simulink model "mesaparasimulink"  (R2017a)
settings: Solver=ode3  StartTime=0.0  StopTime=6.3  FixedStep=5e-3  RelTol=1e-3
undefined symbols (not defined in the file): bloque, bloque1, L1, L2, mesaparasimulink, pasador, RootGround, RootPart
libraries: mblibv1 x24
settings Model: Creator=angel  LastModifiedBy=angel
settings SimMechanicsCC: VisOnUpdateDiagram=on  VisDuringSimulation=on

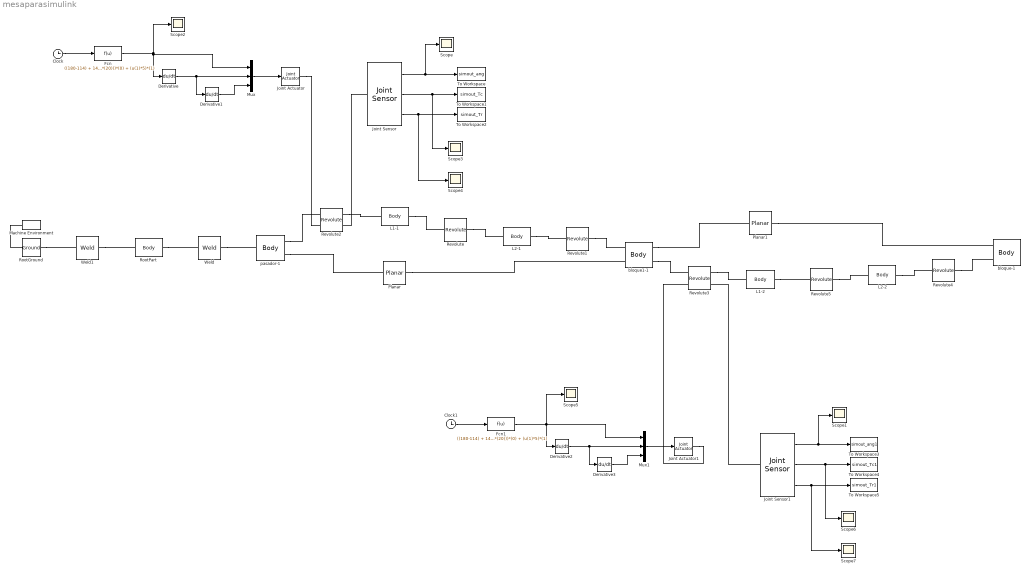
== system mesaparasimulink ==
  Clock : Clock
  Clock1 : Clock
  Derivative{,1..3} (4 alike) : Derivative
  Fcn : Fcn  Expr=((180-114) + 14*sin(2*pi*u(1)*(20)))*(0) + (u(1)*5)*(1)
  Fcn1 : Fcn  Expr=((180-114) + 14*sin(2*pi*u(1)*(20)))*(0) + (u(1)*5)*(1)
  Joint Actuator : mblibv1/Sensors &  Actuators/Joint Actuator  UpdateFromCAD=off  PhysicalDomain=Mechanical  PortType=blob  ActuationStyle=Motion  AngleUnits=rad  ArcVelocityUnits=rad/s  ArcAccelerationUnits=rad/s^2  CoordPositionUnits=m  VelocityUnits=m/s  AccelerationUnits=m/s^2  ForceUnits=N  TorqueUnits=N*m  ActiveIO=on  Width=3  DialogClass=MechanicalActuatorBlock  Primitive=R1  ReferenceFrame=Absolute (World)
      settings: SourceProductName=Simscape Multibody  SourceProductBaseCode=MS
  Joint Actuator1 : mblibv1/Sensors &  Actuators/Joint Actuator  UpdateFromCAD=off  PhysicalDomain=Mechanical  PortType=blob  ActuationStyle=Motion  AngleUnits=rad  ArcVelocityUnits=rad/s  ArcAccelerationUnits=rad/s^2  CoordPositionUnits=m  VelocityUnits=m/s  AccelerationUnits=m/s^2  ForceUnits=N  TorqueUnits=N*m  ActiveIO=on  Width=3  DialogClass=MechanicalActuatorBlock  Primitive=R1  ReferenceFrame=Absolute (World)
      settings: SourceProductName=Simscape Multibody  SourceProductBaseCode=MS
  Joint Sensor : mblibv1/Sensors &  Actuators/Joint Sensor  UpdateFromCAD=off  PhysicalDomain=Mechanical  PortType=blob  Muxed=off  Pose=off  Angle=on  AngleUnits=deg  ArcVelocity=off  ArcVelocityUnits=deg/s  ArcAcceleration=off  ArcAccelerationUnits=deg/s^2  CoordPosition=on  CoordPositionUnits=m  Velocity=off  VelocityUnits=m/s  Acceleration=off  AccelerationUnits=m/s^2  Quaternion=on  QuaternionDT=off  QuaternionDDT=off  QuaternionUnits=off  OutputVector=[1]  ActiveIO=on  Width=5  DialogClass=MechanicalSensorBlock  Primitive=R1  Force=off  ForceUnits=N  Torque=on  TorqueUnits=N*m  ReferenceFrame=Absolute (World)  ReactionSensedSide=Base  ReactionReferenceFrame=Absolute (World)  ReactionForce=off  ReactionForceUnits=N  ReactionMoment=on  ReactionMomentUnits=N*m
      settings: SourceProductName=Simscape Multibody  SourceProductBaseCode=MS
  Joint Sensor1 : mblibv1/Sensors &  Actuators/Joint Sensor  UpdateFromCAD=off  PhysicalDomain=Mechanical  PortType=blob  Muxed=off  Pose=off  Angle=on  AngleUnits=deg  ArcVelocity=off  ArcVelocityUnits=deg/s  ArcAcceleration=off  ArcAccelerationUnits=deg/s^2  CoordPosition=on  CoordPositionUnits=m  Velocity=off  VelocityUnits=m/s  Acceleration=off  AccelerationUnits=m/s^2  Quaternion=on  QuaternionDT=off  QuaternionDDT=off  QuaternionUnits=off  OutputVector=[1]  ActiveIO=on  Width=5  DialogClass=MechanicalSensorBlock  Primitive=R1  Force=off  ForceUnits=N  Torque=on  TorqueUnits=N*m  ReferenceFrame=Absolute (World)  ReactionSensedSide=Base  ReactionReferenceFrame=Absolute (World)  ReactionForce=off  ReactionForceUnits=N  ReactionMoment=on  ReactionMomentUnits=N*m
      settings: SourceProductName=Simscape Multibody  SourceProductBaseCode=MS
  L1-1 : mblibv1/Bodies/Body  LConnTagsString=CS3  RConnTagsString=CS2  UpdateFromCAD=on  PMImportedID=L1-1  DialogClass=MechanicalBodyBlock  Mass=0.00593014  MassUnits=kg  InertiaUnits=kg*m^2  Inertia=[1.04021e-06,0,0;0,1.07865e-06,0;0,0,6.31529e-08]  Shape=Cylinder  ShapeDims=[1 1]  ShapeUnits=m  ShapeUse=false  Density=1  DensityUnits=kg/m^3  DensityUse=false  GraphicsMode=GFXFILE  GraphicsFileName=mesaparasimulink - L1-1.STL  BodyColorSelMode=COLORPALETTE  BodyColor=[0.898039;0.917647;0.929412]  AttachedToCS=CS1  CG=Right$CG$[0.017646 0.00118407 -0.000436433]$WORLD$WORLD$m$[0.521822 0 -0.853055;0 1 0;0.853055 0 0.521822]$3x3 Transform$rad$WORLD$false$L1-1::CG(AUTOGEN)  WorkingFrames=Right$CS1$[0.00058486 -0.00131593 0.01]$WORLD$WORLD$m$[0.521822 0 -0.853055;0 1 0;0.853055 0 0.521822]$3x3 Transform$rad$WORLD$false$L1-1::CS1(AUTOGEN)#Right$CS2$[0.034707 0.00368407 -0.0108729]$WORLD$WORLD$m$[1 0 0;0 1 0;0 0 1]$3x3 Transform$rad$WORLD$true$L1-1:-:L2-1::L1-1(AUTOGEN)#Left$CS3$[0.00058486 0.00368407 0.01]$WORLD$WORLD$m$[1 0 0;0 1 0;0 0 1]$3x3 Transform$rad$WORLD$true$L1-1:-:pasador-1::L1-1(AUTOGEN)  CGPos=[0.017646 0.00118407 -0.000436433]  CGRot=[0.521822 0 -0.853055;0 1 0;0.853055 0 0.521822]  CS0Pos=[]  CS0Rot=[]  CS1Pos=[0.00058486 -0.00131593 0.01]  CS1Rot=[0.521822 0 -0.853055;0 1 0;0.853055 0 0.521822]  CS2Pos=[0.034707 0.00368407 -0.0108729]  CS2Rot=[1 0 0;0 1 0;0 0 1]  CS3Pos=[0.00058486 0.00368407 0.01]  CS3Rot=[1 0 0;0 1 0;0 0 1]  CS4Pos=[]  CS4Rot=[]  CS5Pos=[]  CS5Rot=[]  CS6Pos=[]  CS6Rot=[]  CS7Pos=[]  CS7Rot=[]  CS8Pos=[]  CS8Rot=[]  CS9Pos=[]  CS9Rot=[]  CS10Pos=[]  CS10Rot=[]  CS11Pos=[]  CS11Rot=[]  CS12Pos=[]  CS12Rot=[]  CS13Pos=[]  CS13Rot=[]  CS14Pos=[]  CS14Rot=[]  CS15Pos=[]  CS15Rot=[]  CS16Pos=[]  CS16Rot=[]  CS17Pos=[]  CS17Rot=[]  CS18Pos=[]  CS18Rot=[]  CS19Pos=[]  CS19Rot=[]  CS20Pos=[]  CS20Rot=[]
      settings: SourceProductName=Simscape Multibody  SourceProductBaseCode=MS
  L1-2 : mblibv1/Bodies/Body  LConnTagsString=CS2  RConnTagsString=CS3  UpdateFromCAD=on  PMImportedID=L1-2  DialogClass=MechanicalBodyBlock  Mass=0.00593014  MassUnits=kg  InertiaUnits=kg*m^2  Inertia=[1.04021e-06,0,0;0,1.07865e-06,0;0,0,6.31529e-08]  Shape=Cylinder  ShapeDims=[1 1]  ShapeUnits=m  ShapeUse=false  Density=1  DensityUnits=kg/m^3  DensityUse=false  GraphicsMode=GFXFILE  GraphicsFileName=mesaparasimulink - L1-2.STL  BodyColorSelMode=COLORPALETTE  BodyColor=[0.898039;0.917647;0.929412]  AttachedToCS=CS1  CG=Right$CG$[0.226845 0.0339841 -0.261953]$WORLD$WORLD$m$[0.998014 0 -0.0629932;0 1 0;0.0629932 0 0.998014]$3x3 Transform$rad$WORLD$false$L1-2::CG(AUTOGEN)  WorkingFrames=Right$CS1$[0.225585 0.0314841 -0.241993]$WORLD$WORLD$m$[0.998014 0 -0.0629932;0 1 0;0.0629932 0 0.998014]$3x3 Transform$rad$WORLD$false$L1-2::CS1(AUTOGEN)#Left$CS2$[0.225585 0.0364841 -0.241993]$WORLD$WORLD$m$[1 0 0;0 1 0;0 0 1]$3x3 Transform$rad$WORLD$true$L1-2:-:bloque1-1::L1-2(AUTOGEN)#Right$CS3$[0.228105 0.0364841 -0.281914]$WORLD$WORLD$m$[1 0 0;0 1 0;0 0 1]$3x3 Transform$rad$WORLD$true$L1-2:-:L2-2::L1-2(AUTOGEN)  CGPos=[0.226845 0.0339841 -0.261953]  CGRot=[0.998014 0 -0.0629932;0 1 0;0.0629932 0 0.998014]  CS0Pos=[]  CS0Rot=[]  CS1Pos=[0.225585 0.0314841 -0.241993]  CS1Rot=[0.998014 0 -0.0629932;0 1 0;0.0629932 0 0.998014]  CS2Pos=[0.225585 0.0364841 -0.241993]  CS2Rot=[1 0 0;0 1 0;0 0 1]  CS3Pos=[0.228105 0.0364841 -0.281914]  CS3Rot=[1 0 0;0 1 0;0 0 1]  CS4Pos=[]  CS4Rot=[]  CS5Pos=[]  CS5Rot=[]  CS6Pos=[]  CS6Rot=[]  CS7Pos=[]  CS7Rot=[]  CS8Pos=[]  CS8Rot=[]  CS9Pos=[]  CS9Rot=[]  CS10Pos=[]  CS10Rot=[]  CS11Pos=[]  CS11Rot=[]  CS12Pos=[]  CS12Rot=[]  CS13Pos=[]  CS13Rot=[]  CS14Pos=[]  CS14Rot=[]  CS15Pos=[]  CS15Rot=[]  CS16Pos=[]  CS16Rot=[]  CS17Pos=[]  CS17Rot=[]  CS18Pos=[]  CS18Rot=[]  CS19Pos=[]  CS19Rot=[]  CS20Pos=[]  CS20Rot=[]
      settings: SourceProductName=Simscape Multibody  SourceProductBaseCode=MS
  L2-1 : mblibv1/Bodies/Body  LConnTagsString=CS2  RConnTagsString=CS3  UpdateFromCAD=on  PMImportedID=L2-1  DialogClass=MechanicalBodyBlock  Mass=0.00998014  MassUnits=kg  InertiaUnits=kg*m^2  Inertia=[4.69227e-06,0,0;0,4.75602e-06,0;0,0,1.0534e-07]  Shape=Cylinder  ShapeDims=[1 1]  ShapeUnits=m  ShapeUse=false  Density=1  DensityUnits=kg/m^3  DensityUse=false  GraphicsMode=GFXFILE  GraphicsFileName=mesaparasimulink - L2-1.STL  BodyColorSelMode=COLORPALETTE  BodyColor=[0.898039;0.917647;0.929412]  AttachedToCS=CS1  CG=Right$CG$[0.017646 0.00618407 -0.041433]$WORLD$WORLD$m$[0.873145 0 0.48746;0 1 0;-0.48746 0 0.873145]$3x3 Transform$rad$WORLD$false$L2-1::CG(AUTOGEN)  WorkingFrames=Right$CS1$[0.034707 0.00368407 -0.0108729]$WORLD$WORLD$m$[0.873145 0 0.48746;0 1 0;-0.48746 0 0.873145]$3x3 Transform$rad$WORLD$false$L2-1::CS1(AUTOGEN)#Left$CS2$[0.034707 0.00368407 -0.0108729]$WORLD$WORLD$m$[1 0 0;0 1 0;0 0 1]$3x3 Transform$rad$WORLD$true$L1-1:-:L2-1::L2-1(AUTOGEN)#Right$CS3$[0.00058486 0.00368407 -0.071993]$WORLD$WORLD$m$[1 0 0;0 1 0;0 0 1]$3x3 Transform$rad$WORLD$true$L2-1:-:bloque1-1::L2-1(AUTOGEN)  CGPos=[0.017646 0.00618407 -0.041433]  CGRot=[0.873145 0 0.48746;0 1 0;-0.48746 0 0.873145]  CS0Pos=[]  CS0Rot=[]  CS1Pos=[0.034707 0.00368407 -0.0108729]  CS1Rot=[0.873145 0 0.48746;0 1 0;-0.48746 0 0.873145]  CS2Pos=[0.034707 0.00368407 -0.0108729]  CS2Rot=[1 0 0;0 1 0;0 0 1]  CS3Pos=[0.00058486 0.00368407 -0.071993]  CS3Rot=[1 0 0;0 1 0;0 0 1]  CS4Pos=[]  CS4Rot=[]  CS5Pos=[]  CS5Rot=[]  CS6Pos=[]  CS6Rot=[]  CS7Pos=[]  CS7Rot=[]  CS8Pos=[]  CS8Rot=[]  CS9Pos=[]  CS9Rot=[]  CS10Pos=[]  CS10Rot=[]  CS11Pos=[]  CS11Rot=[]  CS12Pos=[]  CS12Rot=[]  CS13Pos=[]  CS13Rot=[]  CS14Pos=[]  CS14Rot=[]  CS15Pos=[]  CS15Rot=[]  CS16Pos=[]  CS16Rot=[]  CS17Pos=[]  CS17Rot=[]  CS18Pos=[]  CS18Rot=[]  CS19Pos=[]  CS19Rot=[]  CS20Pos=[]  CS20Rot=[]
      settings: SourceProductName=Simscape Multibody  SourceProductBaseCode=MS
  L2-2 : mblibv1/Bodies/Body  LConnTagsString=CS3  RConnTagsString=CS2  UpdateFromCAD=on  PMImportedID=L2-2  DialogClass=MechanicalBodyBlock  Mass=0.00998014  MassUnits=kg  InertiaUnits=kg*m^2  Inertia=[4.69227e-06,0,0;0,4.75602e-06,0;0,0,1.0534e-07]  Shape=Cylinder  ShapeDims=[1 1]  ShapeUnits=m  ShapeUse=false  Density=1  DensityUnits=kg/m^3  DensityUse=false  GraphicsMode=GFXFILE  GraphicsFileName=mesaparasimulink - L2-2.STL  BodyColorSelMode=COLORPALETTE  BodyColor=[0.898039;0.917647;0.929412]  AttachedToCS=CS1  CG=Right$CG$[0.199354 0.0389841 -0.261953]$WORLD$WORLD$m$[-0.570294 0 0.821441;0 1 0;-0.821441 0 -0.570294]$3x3 Transform$rad$WORLD$false$L2-2::CG(AUTOGEN)  WorkingFrames=Right$CS1$[0.228105 0.0364841 -0.281914]$WORLD$WORLD$m$[-0.570294 0 0.821441;0 1 0;-0.821441 0 -0.570294]$3x3 Transform$rad$WORLD$false$L2-2::CS1(AUTOGEN)#Right$CS2$[0.170604 0.0414841 -0.241993]$WORLD$WORLD$m$[1 0 0;0 1 0;0 0 1]$3x3 Transform$rad$WORLD$true$L2-2:-:bloque-1::L2-2(AUTOGEN)#Left$CS3$[0.228105 0.0364841 -0.281914]$WORLD$WORLD$m$[1 0 0;0 1 0;0 0 1]$3x3 Transform$rad$WORLD$true$L1-2:-:L2-2::L2-2(AUTOGEN)  CGPos=[0.199354 0.0389841 -0.261953]  CGRot=[-0.570294 0 0.821441;0 1 0;-0.821441 0 -0.570294]  CS0Pos=[]  CS0Rot=[]  CS1Pos=[0.228105 0.0364841 -0.281914]  CS1Rot=[-0.570294 0 0.821441;0 1 0;-0.821441 0 -0.570294]  CS2Pos=[0.170604 0.0414841 -0.241993]  CS2Rot=[1 0 0;0 1 0;0 0 1]  CS3Pos=[0.228105 0.0364841 -0.281914]  CS3Rot=[1 0 0;0 1 0;0 0 1]  CS4Pos=[]  CS4Rot=[]  CS5Pos=[]  CS5Rot=[]  CS6Pos=[]  CS6Rot=[]  CS7Pos=[]  CS7Rot=[]  CS8Pos=[]  CS8Rot=[]  CS9Pos=[]  CS9Rot=[]  CS10Pos=[]  CS10Rot=[]  CS11Pos=[]  CS11Rot=[]  CS12Pos=[]  CS12Rot=[]  CS13Pos=[]  CS13Rot=[]  CS14Pos=[]  CS14Rot=[]  CS15Pos=[]  CS15Rot=[]  CS16Pos=[]  CS16Rot=[]  CS17Pos=[]  CS17Rot=[]  CS18Pos=[]  CS18Rot=[]  CS19Pos=[]  CS19Rot=[]  CS20Pos=[]  CS20Rot=[]
      settings: SourceProductName=Simscape Multibody  SourceProductBaseCode=MS
  Machine Environment : mblibv1/Bodies/Machine Environment  PortType=env  PhysicalDomain=Mechanical  DialogTemplateClass=MECH.MachineEnvironment  SyncWhenCopied=off  Gravity=[0 -9.81 0]  GravityUnits=m/s^2  GravityAsSignal=off  Dimensionality=Auto-detect  AnalysisType=Forward dynamics  LinearAssemblyTolerance=1e-3  LinearAssemblyToleranceUnits=m  AngularAssemblyTolerance=1e-3  AngularAssemblyToleranceUnits=rad  ConstraintSolverType=Stabilizing  ConstraintRelTolerance=1e-4  ConstraintAbsTolerance=1e-4  UseRobustSingularityHandling=off  RedundancyAnalysisToleranceType=Automatically select tolerance  RedundancyAnalysisTolerance=1e-14  StatePerturbationType=Fixed  PerturbationSize=1e-5  VisualizeMachine=on  BodyVisualizationType=Use model default body geometries  BodyColorSelMode=Use model default  DefaultBodyColor=[1 0 0]
      settings: SourceProductName=Simscape Multibody  SourceProductBaseCode=MS
  Mux : Mux  Inputs=3
  Mux1 : Mux  Inputs=3
  Planar : mblibv1/Joints/Planar  LConnTagsString=__newl0  RConnTagsString=__newr0  UpdateFromCAD=on  PMImportedID=bloque1-1:-:pasador-1  NumSAPorts=0  CutJoint=off  MarkAsCut=off  Primitives=prismatic_prismatic  PrimitiveProps=P1$WORLD$[0,1,0]$prismatic#P2$WORLD$[0,0,1]$prismatic#R1$WORLD$[-1,0,0]$revolute  DialogClass=JointBlock  P1Axis=[0,1,0]  P2Axis=[0,0,1]  R1Axis=[-1,0,0]
      settings: SourceProductName=Simscape Multibody  SourceProductBaseCode=MS
  Planar1 : mblibv1/Joints/Planar  LConnTagsString=__newl0  RConnTagsString=__newr0  UpdateFromCAD=on  PMImportedID=bloque-1:-:bloque1-1  NumSAPorts=0  CutJoint=off  MarkAsCut=off  Primitives=prismatic_prismatic  PrimitiveProps=P1$WORLD$[1,0,0]$prismatic#P2$WORLD$[0,-1,0]$prismatic#R1$WORLD$[0,0,1]$revolute  DialogClass=JointBlock  P1Axis=[1,0,0]  P2Axis=[0,-1,0]  R1Axis=[0,0,1]
      settings: SourceProductName=Simscape Multibody  SourceProductBaseCode=MS
  Revolute : mblibv1/Joints/Revolute  LConnTagsString=__newl0  RConnTagsString=__newr0  UpdateFromCAD=on  PMImportedID=L1-1:-:L2-1  NumSAPorts=0  CutJoint=off  MarkAsCut=off  Primitives=prismatic  PrimitiveProps=R1$WORLD$[0,1,0]$revolute  DialogClass=JointBlock  R1Axis=[0,1,0]
      settings: SourceProductName=Simscape Multibody  SourceProductBaseCode=MS
  Revolute1 : mblibv1/Joints/Revolute  LConnTagsString=__newl0  RConnTagsString=__newr0  UpdateFromCAD=on  PMImportedID=L2-1:-:bloque1-1  NumSAPorts=0  CutJoint=off  MarkAsCut=off  Primitives=prismatic  PrimitiveProps=R1$WORLD$[0,-1,0]$revolute  DialogClass=JointBlock  R1Axis=[0,-1,0]
      settings: SourceProductName=Simscape Multibody  SourceProductBaseCode=MS
  Revolute2 : mblibv1/Joints/Revolute  LConnTagsString=__newl0|SA1  RConnTagsString=__newr0|SA1  UpdateFromCAD=on  PMImportedID=L1-1:-:pasador-1  NumSAPorts=2  CutJoint=off  MarkAsCut=off  Primitives=prismatic  PrimitiveProps=R1$World$[0,-1,0]$revolute  DialogClass=JointBlock  R1Axis=[0,-1,0]
      settings: SourceProductName=Simscape Multibody  SourceProductBaseCode=MS
  Revolute3 : mblibv1/Joints/Revolute  LConnTagsString=__newl0|SA1  RConnTagsString=__newr0|SA1  UpdateFromCAD=on  PMImportedID=L1-2:-:bloque1-1  NumSAPorts=2  CutJoint=off  MarkAsCut=off  Primitives=prismatic  PrimitiveProps=R1$World$[0,-1,0]$revolute  DialogClass=JointBlock  R1Axis=[0,-1,0]
      settings: SourceProductName=Simscape Multibody  SourceProductBaseCode=MS
  Revolute4 : mblibv1/Joints/Revolute  LConnTagsString=__newl0  RConnTagsString=__newr0  UpdateFromCAD=on  PMImportedID=L2-2:-:bloque-1  NumSAPorts=0  CutJoint=off  MarkAsCut=off  Primitives=prismatic  PrimitiveProps=R1$WORLD$[0,-1,0]$revolute  DialogClass=JointBlock  R1Axis=[0,-1,0]
      settings: SourceProductName=Simscape Multibody  SourceProductBaseCode=MS
  Revolute5 : mblibv1/Joints/Revolute  LConnTagsString=__newl0  RConnTagsString=__newr0  UpdateFromCAD=on  PMImportedID=L1-2:-:L2-2  NumSAPorts=0  CutJoint=off  MarkAsCut=off  Primitives=prismatic  PrimitiveProps=R1$WORLD$[0,1,0]$revolute  DialogClass=JointBlock  R1Axis=[0,1,0]
      settings: SourceProductName=Simscape Multibody  SourceProductBaseCode=MS
  RootGround : mblibv1/Bodies/Ground  UpdateFromCAD=on  PMImportedID=RootGround  LeftPortType=env  RightPortType=workingframe  PhysicalDomain=Mechanical  DialogClass=GroundBlock  CoordPosition=[0.0155003,0.0188998,-0.240245]  CoordPositionUnits=m  StateVectorMgrId=2  MachineId=[3 0]  ShowEnvPort=on  ParameterChecksum=[2085027060, 2068719643, 829486895, 247911722]  TopologyChecksum=[3575472688, 637684525, 4187757033, 1155351781]
      settings: SourceProductName=Simscape Multibody  SourceProductBaseCode=MS
  RootPart : mblibv1/Bodies/Body  LConnTagsString=CS3  RConnTagsString=CS2  UpdateFromCAD=on  PMImportedID=mesaparasimulink/RootPart  DialogClass=MechanicalBodyBlock  Mass=0  MassUnits=kg  InertiaUnits=kg*m^2  Inertia=[0,0,0;0,0,0;0,0,0]  Shape=Cylinder  ShapeDims=[1 1]  ShapeUnits=m  ShapeUse=false  Density=1  DensityUnits=kg/m^3  DensityUse=false  GraphicsMode=MACHINE_DEFAULT  BodyColorSelMode=MACHINE_DEFAULT  BodyColor=[1;0;0]  AttachedToCS=CS1  CG=Right$CG$[0.0155003 0.0188998 -0.240245]$WORLD$WORLD$m$[1 0 0;0 1 0;0 0 1]$3x3 Transform$rad$WORLD$false$mesaparasimulink/RootPart::CG(AUTOGEN)  WorkingFrames=Right$CS1$[0 0 0]$WORLD$WORLD$m$[1 0 0;0 1 0;0 0 1]$3x3 Transform$rad$WORLD$false$mesaparasimulink/RootPart::CS1(AUTOGEN)#Right$CS2$[0.015217 0.00611225 -0.044476]$WORLD$WORLD$m$[1 0 0;0 1 0;0 0 1]$3x3 Transform$rad$WORLD$true$mesaparasimulink/RootPart:-:pasador-1::mesaparasimulink/RootPart(AUTOGEN)#Left$CS3$[0.0155003 0.0188998 -0.240245]$WORLD$WORLD$m$[1 0 0;0 1 0;0 0 1]$3x3 Transform$rad$WORLD$true$RootGround:-:mesaparasimulink/RootPart::mesaparasimulink/RootPart(AUTOGEN)  CGPos=[0.0155003 0.0188998 -0.240245]  CGRot=[1 0 0;0 1 0;0 0 1]  CS0Pos=[]  CS0Rot=[]  CS1Pos=[0 0 0]  CS1Rot=[1 0 0;0 1 0;0 0 1]  CS2Pos=[0.015217 0.00611225 -0.044476]  CS2Rot=[1 0 0;0 1 0;0 0 1]  CS3Pos=[0.0155003 0.0188998 -0.240245]  CS3Rot=[1 0 0;0 1 0;0 0 1]  CS4Pos=[]  CS4Rot=[]  CS5Pos=[]  CS5Rot=[]  CS6Pos=[]  CS6Rot=[]  CS7Pos=[]  CS7Rot=[]  CS8Pos=[]  CS8Rot=[]  CS9Pos=[]  CS9Rot=[]  CS10Pos=[]  CS10Rot=[]  CS11Pos=[]  CS11Rot=[]  CS12Pos=[]  CS12Rot=[]  CS13Pos=[]  CS13Rot=[]  CS14Pos=[]  CS14Rot=[]  CS15Pos=[]  CS15Rot=[]  CS16Pos=[]  CS16Rot=[]  CS17Pos=[]  CS17Rot=[]  CS18Pos=[]  CS18Rot=[]  CS19Pos=[]  CS19Rot=[]  CS20Pos=[]  CS20Rot=[]
      settings: SourceProductName=Simscape Multibody  SourceProductBaseCode=MS
  Scope{,1..7} (8 alike) : Scope
  To Workspace : ToWorkspace  VariableName=simout_ang  SaveFormat=Timeseries  SampleTime=-1
  To Workspace1 : ToWorkspace  VariableName=simout_Tc  SaveFormat=Timeseries  SampleTime=-1
  To Workspace2 : ToWorkspace  VariableName=simout_Tr  SaveFormat=Timeseries  SampleTime=-1
  To Workspace3 : ToWorkspace  VariableName=simout_ang1  SaveFormat=Timeseries  SampleTime=-1
  To Workspace4 : ToWorkspace  VariableName=simout_Tc1  SaveFormat=Timeseries  SampleTime=-1
  To Workspace5 : ToWorkspace  VariableName=simout_Tr1  SaveFormat=Timeseries  SampleTime=-1
  Weld : mblibv1/Joints/Weld  LConnTagsString=__newl0  RConnTagsString=__newr0  UpdateFromCAD=on  PMImportedID=mesaparasimulink/RootPart:-:pasador-1  NumSAPorts=0  CutJoint=off  MarkAsCut=off  Primitives=weld  PrimitiveProps=W$WORLD$[0.57735,0.57735,0.57735]$weld  DialogClass=JointBlock  WAxis=[0.57735,0.57735,0.57735]
      settings: SourceProductName=Simscape Multibody  SourceProductBaseCode=MS
  Weld1 : mblibv1/Joints/Weld  LConnTagsString=__newl0  RConnTagsString=__newr0  UpdateFromCAD=on  PMImportedID=RootGround:-:mesaparasimulink/RootPart  NumSAPorts=0  CutJoint=off  MarkAsCut=off  Primitives=weld  PrimitiveProps=W$WORLD$[0.57735,0.57735,0.57735]$weld  DialogClass=JointBlock  WAxis=[0.57735,0.57735,0.57735]
      settings: SourceProductName=Simscape Multibody  SourceProductBaseCode=MS
  bloque-1 : mblibv1/Bodies/Body  LConnTagsString=CS2|CS3  UpdateFromCAD=on  PMImportedID=bloque-1  DialogClass=MechanicalBodyBlock  Mass=1.38082  MassUnits=kg  InertiaUnits=kg*m^2  Inertia=[0.0207014,0,0;0,0.0416806,0;0,0,0.0211297]  Shape=Cylinder  ShapeDims=[1 1]  ShapeUnits=m  ShapeUse=false  Density=1  DensityUnits=kg/m^3  DensityUse=false  GraphicsMode=GFXFILE  GraphicsFileName=mesaparasimulink - bloque-1.STL  BodyColorSelMode=COLORPALETTE  BodyColor=[0.647059;0.619608;0.588235]  AttachedToCS=CS1  CG=Right$CG$[0.00249192 0.0389841 -0.241993]$WORLD$WORLD$m$[1 0 0;0 1 0;0 0 1]$3x3 Transform$rad$WORLD$false$bloque-1::CG(AUTOGEN)  WorkingFrames=Right$CS1$[0.000603728 0.0389841 -0.241993]$WORLD$WORLD$m$[1 0 0;0 1 0;0 0 1]$3x3 Transform$rad$WORLD$false$bloque-1::CS1(AUTOGEN)#Left$CS2$[0.129445 0.0614841 -0.246993]$WORLD$WORLD$m$[1 0 0;0 1 0;0 0 1]$3x3 Transform$rad$WORLD$true$bloque-1:-:bloque1-1::bloque-1(AUTOGEN)#Left$CS3$[0.170604 0.0414841 -0.241993]$WORLD$WORLD$m$[1 0 0;0 1 0;0 0 1]$3x3 Transform$rad$WORLD$true$L2-2:-:bloque-1::bloque-1(AUTOGEN)  CGPos=[0.00249192 0.0389841 -0.241993]  CGRot=[1 0 0;0 1 0;0 0 1]  CS0Pos=[]  CS0Rot=[]  CS1Pos=[0.000603728 0.0389841 -0.241993]  CS1Rot=[1 0 0;0 1 0;0 0 1]  CS2Pos=[0.129445 0.0614841 -0.246993]  CS2Rot=[1 0 0;0 1 0;0 0 1]  CS3Pos=[0.170604 0.0414841 -0.241993]  CS3Rot=[1 0 0;0 1 0;0 0 1]  CS4Pos=[]  CS4Rot=[]  CS5Pos=[]  CS5Rot=[]  CS6Pos=[]  CS6Rot=[]  CS7Pos=[]  CS7Rot=[]  CS8Pos=[]  CS8Rot=[]  CS9Pos=[]  CS9Rot=[]  CS10Pos=[]  CS10Rot=[]  CS11Pos=[]  CS11Rot=[]  CS12Pos=[]  CS12Rot=[]  CS13Pos=[]  CS13Rot=[]  CS14Pos=[]  CS14Rot=[]  CS15Pos=[]  CS15Rot=[]  CS16Pos=[]  CS16Rot=[]  CS17Pos=[]  CS17Rot=[]  CS18Pos=[]  CS18Rot=[]  CS19Pos=[]  CS19Rot=[]  CS20Pos=[]  CS20Rot=[]
      settings: SourceProductName=Simscape Multibody  SourceProductBaseCode=MS
  bloque1-1 : mblibv1/Bodies/Body  LConnTagsString=CS2|CS3  RConnTagsString=CS4|CS5  UpdateFromCAD=on  PMImportedID=bloque1-1  DialogClass=MechanicalBodyBlock  Mass=2.30927 + (0.7)*(1)  MassUnits=kg  InertiaUnits=kg*m^2  Inertia=[0.0339371,-0.000140996,-0.000492128;-0.000140996,0.0550496,-0.00133315;-0.000492128,-0.00133315,0.0222148]  Shape=Cylinder  ShapeDims=[1 1]  ShapeUnits=m  ShapeUse=false  Density=1  DensityUnits=kg/m^3  DensityUse=false  GraphicsMode=GFXFILE  GraphicsFileName=mesaparasimulink - bloque1-1.STL  BodyColorSelMode=COLORPALETTE  BodyColor=[0.64706 0.61961 0.58823]  AttachedToCS=CS1  CG=Right$CG$[0.021929 0.006979 -0.242263]$WORLD$WORLD$m$[0 0 1;0 1 0;-1 0 0]$3x3 Transform$rad$WORLD$false$bloque1-1::CG(AUTOGEN)  WorkingFrames=Right$CS1$[0.00058486 0.00618407 -0.241993]$WORLD$WORLD$m$[0 0 1;0 1 0;-1 0 0]$3x3 Transform$rad$WORLD$false$bloque1-1::CS1(AUTOGEN)#Left$CS2$[0.00058486 0.00368407 -0.071993]$WORLD$WORLD$m$[1 0 0;0 1 0;0 0 1]$3x3 Transform$rad$WORLD$true$L2-1:-:bloque1-1::bloque1-1(AUTOGEN)#Left$CS3$[0.00558486 0.0186841 -0.0657822]$WORLD$WORLD$m$[1 0 0;0 1 0;0 0 1]$3x3 Transform$rad$WORLD$true$bloque1-1:-:pasador-1::bloque1-1(AUTOGEN)#Right$CS4$[0.129445 0.0614841 -0.246993]$WORLD$WORLD$m$[1 0 0;0 1 0;0 0 1]$3x3 Transform$rad$WORLD$true$bloque-1:-:bloque1-1::bloque1-1(AUTOGEN)#Right$CS5$[0.225585 0.0364841 -0.241993]$WORLD$WORLD$m$[1 0 0;0 1 0;0 0 1]$3x3 Transform$rad$WORLD$true$L1-2:-:bloque1-1::bloque1-1(AUTOGEN)  CGPos=[0.021929 0.006979 -0.242263]  CGRot=[0 0 1;0 1 0;-1 0 0]  CS0Pos=[]  CS0Rot=[]  CS1Pos=[0.00058486 0.00618407 -0.241993]  CS1Rot=[0 0 1;0 1 0;-1 0 0]  CS2Pos=[0.00058486 0.00368407 -0.071993]  CS2Rot=[1 0 0;0 1 0;0 0 1]  CS3Pos=[0.00558486 0.0186841 -0.0657822]  CS3Rot=[1 0 0;0 1 0;0 0 1]  CS4Pos=[0.129445 0.0614841 -0.246993]  CS4Rot=[1 0 0;0 1 0;0 0 1]  CS5Pos=[0.225585 0.0364841 -0.241993]  CS5Rot=[1 0 0;0 1 0;0 0 1]  CS6Pos=[]  CS6Rot=[]  CS7Pos=[]  CS7Rot=[]  CS8Pos=[]  CS8Rot=[]  CS9Pos=[]  CS9Rot=[]  CS10Pos=[]  CS10Rot=[]  CS11Pos=[]  CS11Rot=[]  CS12Pos=[]  CS12Rot=[]  CS13Pos=[]  CS13Rot=[]  CS14Pos=[]  CS14Rot=[]  CS15Pos=[]  CS15Rot=[]  CS16Pos=[]  CS16Rot=[]  CS17Pos=[]  CS17Rot=[]  CS18Pos=[]  CS18Rot=[]  CS19Pos=[]  CS19Rot=[]  CS20Pos=[]  CS20Rot=[]
      settings: SourceProductName=Simscape Multibody  SourceProductBaseCode=MS
  pasador-1 : mblibv1/Bodies/Body  LConnTagsString=CS2  RConnTagsString=CS3|CS4  UpdateFromCAD=on  PMImportedID=pasador-1  DialogClass=MechanicalBodyBlock  Mass=0.0205054  MassUnits=kg  InertiaUnits=kg*m^2  Inertia=[4.58203e-06,-2.15476e-08,1.58023e-07;-2.15476e-08,4.20111e-06,8.02226e-08;1.58023e-07,8.02226e-08,1.75975e-06]  Shape=Cylinder  ShapeDims=[1 1]  ShapeUnits=m  ShapeUse=false  Density=1  DensityUnits=kg/m^3  DensityUse=false  GraphicsMode=GFXFILE  GraphicsFileName=mesaparasimulink - pasador-1.STL  BodyColorSelMode=COLORPALETTE  BodyColor=[0.792157;0.819608;0.933333]  AttachedToCS=CS1  CG=Right$CG$[0.015217 0.00611225 -0.044476]$WORLD$WORLD$m$[1 0 0;0 1 0;0 0 1]$3x3 Transform$rad$WORLD$false$pasador-1::CG(AUTOGEN)  WorkingFrames=Right$CS1$[0.00058486 -0.00631593 0.01]$WORLD$WORLD$m$[1 0 0;0 1 0;0 0 1]$3x3 Transform$rad$WORLD$false$pasador-1::CS1(AUTOGEN)#Left$CS2$[0.015217 0.00611225 -0.044476]$WORLD$WORLD$m$[1 0 0;0 1 0;0 0 1]$3x3 Transform$rad$WORLD$true$mesaparasimulink/RootPart:-:pasador-1::pasador-1(AUTOGEN)#Right$CS3$[0.00058486 0.00368407 0.01]$WORLD$WORLD$m$[1 0 0;0 1 0;0 0 1]$3x3 Transform$rad$WORLD$true$L1-1:-:pasador-1::pasador-1(AUTOGEN)#Right$CS4$[0.00558486 0.0186841 -0.0657822]$WORLD$WORLD$m$[1 0 0;0 1 0;0 0 1]$3x3 Transform$rad$WORLD$true$bloque1-1:-:pasador-1::pasador-1(AUTOGEN)  CGPos=[0.015217 0.00611225 -0.044476]  CGRot=[1 0 0;0 1 0;0 0 1]  CS0Pos=[]  CS0Rot=[]  CS1Pos=[0.00058486 -0.00631593 0.01]  CS1Rot=[1 0 0;0 1 0;0 0 1]  CS2Pos=[0.015217 0.00611225 -0.044476]  CS2Rot=[1 0 0;0 1 0;0 0 1]  CS3Pos=[0.00058486 0.00368407 0.01]  CS3Rot=[1 0 0;0 1 0;0 0 1]  CS4Pos=[0.00558486 0.0186841 -0.0657822]  CS4Rot=[1 0 0;0 1 0;0 0 1]  CS5Pos=[]  CS5Rot=[]  CS6Pos=[]  CS6Rot=[]  CS7Pos=[]  CS7Rot=[]  CS8Pos=[]  CS8Rot=[]  CS9Pos=[]  CS9Rot=[]  CS10Pos=[]  CS10Rot=[]  CS11Pos=[]  CS11Rot=[]  CS12Pos=[]  CS12Rot=[]  CS13Pos=[]  CS13Rot=[]  CS14Pos=[]  CS14Rot=[]  CS15Pos=[]  CS15Rot=[]  CS16Pos=[]  CS16Rot=[]  CS17Pos=[]  CS17Rot=[]  CS18Pos=[]  CS18Rot=[]  CS19Pos=[]  CS19Rot=[]  CS20Pos=[]  CS20Rot=[]
      settings: SourceProductName=Simscape Multibody  SourceProductBaseCode=MS
  wires:
  Clock/1 -> Fcn/1
  Mux/1 -> Joint Actuator/1
  Fcn/1 -> Derivative/1, Mux/1, Scope2/1
  Joint Sensor/3 -> Scope4/1, To Workspace2/1
  Derivative/1 -> Derivative1/1, Mux/2
  Joint Sensor/2 -> Scope3/1, To Workspace1/1
  Derivative1/1 -> Mux/3
  Joint Sensor/1 -> Scope/1, To Workspace/1
  Clock1/1 -> Fcn1/1
  Mux1/1 -> Joint Actuator1/1
  Fcn1/1 -> Derivative2/1, Mux1/1, Scope5/1
  Joint Sensor1/3 -> Scope7/1, To Workspace5/1
  Derivative2/1 -> Derivative3/1, Mux1/2
  Joint Sensor1/2 -> Scope6/1, To Workspace4/1
  Derivative3/1 -> Mux1/3
  Joint Sensor1/1 -> Scope1/1, To Workspace3/1
  connections:
  RootPart/RConn1 -- Weld/LConn1
  Weld/RConn1 -- pasador-1/LConn1
  L1-1/RConn1 -- Revolute/LConn1
  Revolute/RConn1 -- L2-1/LConn1
  L2-1/RConn1 -- Revolute1/LConn1
  Revolute1/RConn1 -- bloque1-1/LConn1
  pasador-1/RConn1 -- Revolute2/LConn1
  Revolute2/RConn1 -- L1-1/LConn1
  pasador-1/RConn2 -- Planar/LConn1
  Planar/RConn1 -- bloque1-1/LConn2
  bloque1-1/RConn1 -- Planar1/LConn1
  Planar1/RConn1 -- bloque-1/LConn1
  bloque1-1/RConn2 -- Revolute3/LConn1
  Revolute3/RConn1 -- L1-2/LConn1
  L2-2/RConn1 -- Revolute4/LConn1
  Revolute4/RConn1 -- bloque-1/LConn2
  L1-2/RConn1 -- Revolute5/LConn1
  Revolute5/RConn1 -- L2-2/LConn1
  RootGround/RConn1 -- Weld1/LConn1
  Weld1/RConn1 -- RootPart/LConn1
  RootGround/LConn1 -- Machine Environment/RConn1
  Joint Actuator/RConn1 -- Revolute2/LConn2
  Joint Sensor/LConn1 -- Revolute2/RConn2
  Joint Actuator1/RConn1 -- Revolute3/LConn2
  Joint Sensor1/LConn1 -- Revolute3/RConn2
